simulink model "bicyclemodel_sinusoid_simulation"  (R2014b)
settings: Solver=ode45  StartTime=0.0  StopTime=60  RelTol=1e-3
settings Model: Creator=wangze  LastModifiedBy=wangze
settings DataIOCC: LimitDataPoints=off
settings OptimizationCC: UseDivisionForNetSlopeComputation=off  SimCompilerOptimization=off
settings DebuggingCC: FrameProcessingCompatibilityMsg=error  AllowSymbolicDim=off
settings RTWCC: RTWCompilerOptimization=off
settings ConfigComp: CovMetricSettings=dw  CovHtmlReporting=on  CovSaveCumulativeToWorkspaceVar=on  CovSaveSingleToWorkspaceVar=on  CovModelRefEnable=Off  CovExternalEMLEnable=off  CovSFcnEnable=off

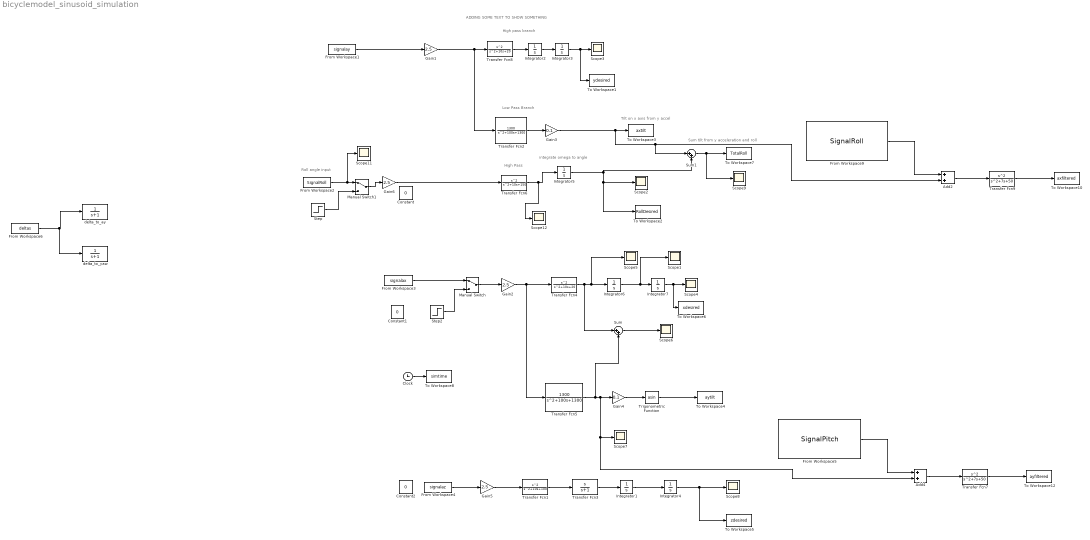
== system bicyclemodel_sinusoid_simulation ==
  note: integrate omega to angle
  note: ADDING SOME TEXT TO SHOW SOMETHING
  note: Roll angle input
  note: Tilt on x axis from y accel
  note: Sum tilt from y acceleration and roll
  note: High Pass
  note: Low Pass Branch
  note: High pass branch
  Add2 : Sum
  Add4 : Sum
  Clock : Clock
  Constant : Constant  Value=0
  Constant1 : Constant  Value=0
  Constant2 : Constant  Value=0
  From Workspace1 : FromWorkspace  VariableName=signalay  SampleTime=0.05
  From Workspace2 : FromWorkspace  VariableName=SignalRoll  SampleTime=0.05
  From Workspace3 : FromWorkspace  VariableName=signalax  SampleTime=0.05
  From Workspace4 : FromWorkspace  VariableName=signalaz  SampleTime=0.05
  From Workspace5 : FromWorkspace  VariableName=SignalPitch  SampleTime=0
  From Workspace6 : FromWorkspace  VariableName=deltas  SampleTime=0.05
  From Workspace9 : FromWorkspace  VariableName=SignalRoll  SampleTime=0
  Gain{1..2,5..6} (4 alike) : Gain  Gain=2.5  SampleTime=0.05
  Gain3 : Gain  Gain=0.1  SampleTime=0.05
  Gain4 : Gain  Gain=0.1  SampleTime=0.05
  Integrator{1..7} (7 alike) : Integrator
  Manual Switch : ManualSwitch
  Manual Switch1 : ManualSwitch
  Scope{1..9,11..12} (11 alike) : Scope
      Scope1 settings: YMin=-0.28187  YMax=0.50005
      Scope11 settings: SaveName=ScopeData8
      Scope12 settings: SaveName=ScopeData9
      Scope4 settings: YMin=-0.02978  YMax=0.19107  SaveName=ScopeData4
      Scope5 settings: YMin=-4.15952  YMax=4.62545  SaveName=ScopeData5
      Scope6 settings: YMin=-1.35826  YMax=8.01741  SaveName=ScopeData6
      Scope7 settings: YMin=-0.67403  YMax=4.06297  SaveName=ScopeData7
      Scope9 settings: SaveName=ScopeData2
  Step : Step  SampleTime=0
  Step2 : Step  Time=0  SampleTime=0
  Sum : Sum  Inputs=|++
  Sum1 : Sum  Inputs=|++
  To Workspace1 : ToWorkspace  VariableName=ydesired  SampleTime=0.05
      settings: Decimation=2  Save2DSignal=2-D array (concatenate along first dimension)
  To Workspace10 : ToWorkspace  VariableName=axfiltered  SampleTime=-1
  To Workspace12 : ToWorkspace  VariableName=ayfiltered  SampleTime=-1
  To Workspace2 : ToWorkspace  VariableName=RollDesired  SampleTime=0.05
      settings: Decimation=2
  To Workspace3 : ToWorkspace  VariableName=axtilt  SampleTime=0.05
      settings: Decimation=2  Save2DSignal=2-D array (concatenate along first dimension)
  To Workspace4 : ToWorkspace  VariableName=aytilt  SampleTime=0.05
      settings: Decimation=2  Save2DSignal=2-D array (concatenate along first dimension)
  To Workspace5 : ToWorkspace  VariableName=zdesired  SampleTime=0.05
      settings: Decimation=2
  To Workspace6 : ToWorkspace  VariableName=xdesired  SampleTime=0.05
      settings: Decimation=2  Save2DSignal=2-D array (concatenate along first dimension)
  To Workspace7 : ToWorkspace  VariableName=TotalRoll  SampleTime=0.05
      settings: Decimation=2  Save2DSignal=2-D array (concatenate along first dimension)
  To Workspace8 : ToWorkspace  VariableName=simtime  SampleTime=-1
      settings: Decimation=2  Save2DSignal=2-D array (concatenate along first dimension)
  Transfer Fcn1 : TransferFcn  Numerator=[1 0 0]  Denominator=[1 10 100]
  Transfer Fcn2 : TransferFcn  Numerator=[1300]  Denominator=[1 100 1300]
  Transfer Fcn3 : TransferFcn  Numerator=[1 0]  Denominator=[1 1]
  Transfer Fcn4 : TransferFcn  Numerator=[1 0 0]  Denominator=[1 10 20]
  Transfer Fcn5 : TransferFcn  Numerator=[1300]  Denominator=[1 100 1300]
  Transfer Fcn6 : TransferFcn  Numerator=[1 0 0]  Denominator=[1 10 150]
  Transfer Fcn7 : TransferFcn  Numerator=[1 0 0]  Denominator=[1 7 50]
  Transfer Fcn8 : TransferFcn  Numerator=[1 0 0]  Denominator=[1 10 20]
  Transfer Fcn9 : TransferFcn  Numerator=[1 0 0]  Denominator=[1 7 50]
  Trigonometric Function : Trigonometry  Operator=asin
  delta_to_ay : TransferFcn  Denominator=[1 1]
  delta_to_yaw : TransferFcn  Denominator=[1 1]
  wires:
  Integrator2/1 -> Integrator3/1
  Integrator3/1 -> Scope3/1, To Workspace1/1
  Integrator6/1 -> Scope1/1, Integrator7/1
  Transfer Fcn4/1 -> Sum/1, Scope5/1, Integrator6/1
  Integrator7/1 -> To Workspace6/1, Scope4/1
  Gain1/1 -> Transfer Fcn2/1, Transfer Fcn8/1
  Gain4/1 -> Trigonometric Function/1
  Transfer Fcn5/1 -> Sum/2, Add4/2, Scope7/1, Gain4/1
  Gain2/1 -> Transfer Fcn5/1, Transfer Fcn4/1
  Manual Switch/1 -> Gain2/1
  From Workspace1/1 -> Gain1/1
  Transfer Fcn8/1 -> Integrator2/1
  From Workspace4/1 -> Gain5/1
  Gain5/1 -> Transfer Fcn1/1
  Transfer Fcn1/1 -> Transfer Fcn3/1
  Transfer Fcn3/1 -> Integrator1/1
  Integrator1/1 -> Integrator4/1
  Integrator4/1 -> To Workspace5/1, Scope8/1
  Step2/1 -> Manual Switch/2
  From Workspace3/1 -> Manual Switch/1
  Sum/1 -> Scope6/1
  Transfer Fcn2/1 -> Gain3/1
  Trigonometric Function/1 -> To Workspace4/1
  Clock/1 -> To Workspace8/1
  Gain3/1 -> Add2/2, Sum1/1, To Workspace3/1
  Sum1/1 -> Scope9/1, To Workspace7/1
  From Workspace2/1 -> Scope11/1, Manual Switch1/1
  Manual Switch1/1 -> Gain6/1
  Step/1 -> Manual Switch1/2
  Gain6/1 -> Transfer Fcn6/1
  Transfer Fcn6/1 -> Scope12/1, Integrator5/1
  Integrator5/1 -> Sum1/2, To Workspace2/1, Scope2/1
  From Workspace5/1 -> Add4/1
  Add4/1 -> Transfer Fcn7/1
  Transfer Fcn7/1 -> To Workspace12/1
  From Workspace9/1 -> Add2/1
  Add2/1 -> Transfer Fcn9/1
  Transfer Fcn9/1 -> To Workspace10/1
  From Workspace6/1 -> delta_to_yaw/1, delta_to_ay/1
